simulink model "Regulateur_Proportionel_Integrale_Derive_Zeigler_Nicole"  (R2017a)
settings: Solver=VariableStepAuto  StartTime=0.0  StopTime=20  RelTol=1e-3
values from neighbouring files (symbols this model uses):
  Kp = 1.2 * T / L    (= 18)    [declaration_des_variables.m]
  Ti = 2 * L    (= 0.4)    [declaration_des_variables.m]
settings Model: Creator=PC  LastModifiedBy=PC

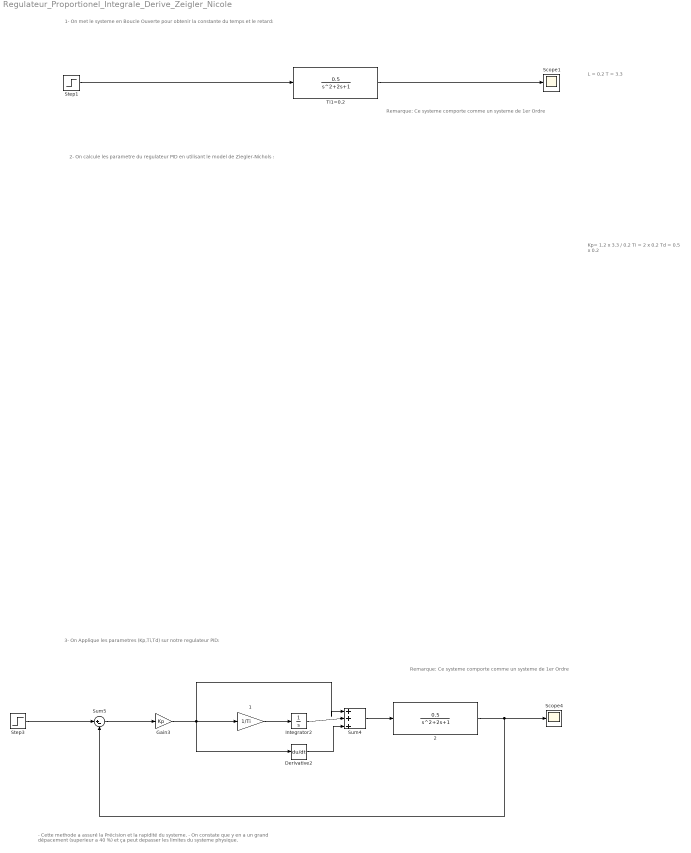
== system Regulateur_Proportionel_Integrale_Derive_Zeigler_Nicole ==
  note: Remarque: Ce systeme comporte comme
      | un systeme de 1er Ordre
  note: - Cette methode a assuré la Précision et la rapidité du systeme.
      | - On constate que y en a un grand dépacement (superieur a 40 %) et ça peut depasser les limites du systeme physique.
  note: L = 0.2
      | T = 3.3
  note: 2- On calcule les parametre du regulateur PID en utilisant le model de Ziegler-Nichols :
  note: 1- On met le systeme en Boucle Ouverte pour obtenir la constante du temps et le retard:
  note: Kp= 1.2 x 3.3 / 0.2
      | Ti = 2 x 0.2
      | Td = 0.5 x 0.2
  note: 3- On Applique les parametres (Kp,Ti,Td) sur notre regulateur PID:
  note: Remarque: Ce systeme comporte comme
      | un systeme de 1er Ordre
  "1 " : Gain  Gain=1/Ti
  2 : TransferFcn  Numerator=[0.5]
  Derivative2 : Derivative  CoefficientInTFapproximation=Td
  Gain3 : Gain  Gain=Kp
  Integrator2 : Integrator
  Scope1 : Scope
  Scope4 : Scope
  Step1 : Step  Time=0  SampleTime=0
  Step3 : Step  Time=0  SampleTime=0
  Sum4 : Sum  Inputs=|+++
  Sum5 : Sum  Inputs=|+-
  Ti1=0.2 : TransferFcn  Numerator=[0.5]
  wires:
  Ti1=0.2/1 -> Scope1/1
  Step1/1 -> Ti1=0.2/1
  Gain3/1 -> "1 "/1, Sum4/1, Derivative2/1
  2/1 -> Sum5/2, Scope4/1
  Sum4/1 -> 2/1
  Derivative2/1 -> Sum4/3
  Integrator2/1 -> Sum4/2
  Sum5/1 -> Gain3/1
  "1 "/1 -> Integrator2/1
  Step3/1 -> Sum5/1
